simulink library "INT_Tra_TrqRed"  (R2016b)
settings: Solver=VariableStepAuto  StartTime=0.0  StopTime=10.0  RelTol=1e-3
settings Model: Creator=lenovo  LastModifiedBy=lenovo

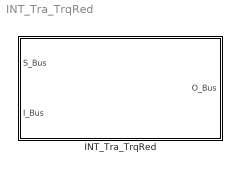
== system INT_Tra_TrqRed ==
  INT_Tra_TrqRed : Subsystem

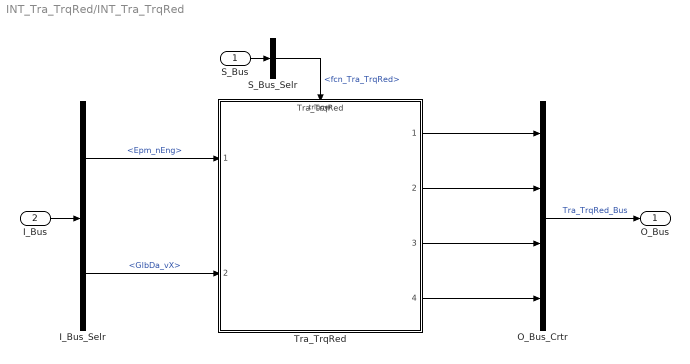
== system INT_Tra_TrqRed/INT_Tra_TrqRed ==
  S_Bus : Inport
  I_Bus : Inport  Port=2
  I_Bus_Selr : BusSelector  OutputSignals=Epm_nEng,GlbDa_vX
  O_Bus_Crtr : BusCreator  Inputs=4
  S_Bus_Selr : BusSelector  OutputSignals=fcn_Tra_TrqRed
  Tra_TrqRed : ModelReference  ModelNameDialog=Tra_TrqRed  SimulationMode=Normal  ModelReferenceVersion=1.4  TriggerPortName=function  TriggerPortTriggerType=function-call  TriggerPortStatesWhenEnabling=held
  O_Bus : Outport
  wires:
  S_Bus_Selr/1 -> Tra_TrqRed/Trigger  "<fcn_Tra_TrqRed>"
  S_Bus/1 -> S_Bus_Selr/1
  I_Bus/1 -> I_Bus_Selr/1
  I_Bus_Selr/1 -> Tra_TrqRed/1  "<Epm_nEng>"
  I_Bus_Selr/2 -> Tra_TrqRed/2  "<GlbDa_vX>"
  O_Bus_Crtr/1 -> O_Bus/1  "Tra_TrqRed_Bus"
  Tra_TrqRed/1 -> O_Bus_Crtr/1
  Tra_TrqRed/2 -> O_Bus_Crtr/2
  Tra_TrqRed/3 -> O_Bus_Crtr/3
  Tra_TrqRed/4 -> O_Bus_Crtr/4
